simulink model "turtlebot"  (R2023b)
settings: Solver=VariableStepAuto  StartTime=0.0  StopTime=35  RelTol=1e-3
values from neighbouring files (symbols this model uses):
  A = [-2*xcarthography' -2*ycarthography' ones(N,1)]    [circle_linear_regression.m]    (also in turtlebot_sim.m = [r/2 r/2; r/d -r/d])
  Ki = 0.47    [turtlebot_sim.m]
  Kp = 1.2    [turtlebot_sim.m]
  Ts = 0.1    [turtlebot_sim.m]
  x0 = X(1)    [circle_linear_regression.m]    (also in turtlebot_sim.m = [0 0 0])
libraries: slpidlib x2
settings Model: Creator=reda

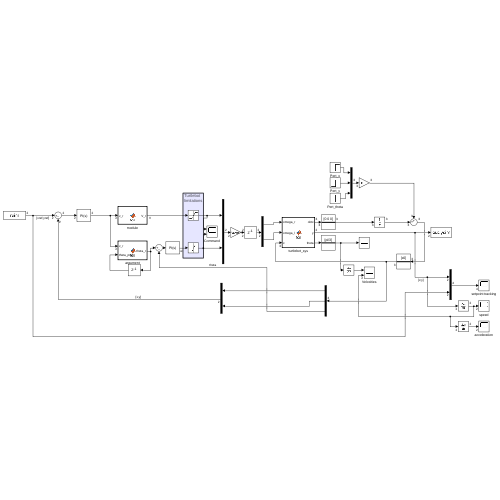
[thumbnail: Simulink's stored preview of the top-level diagram]
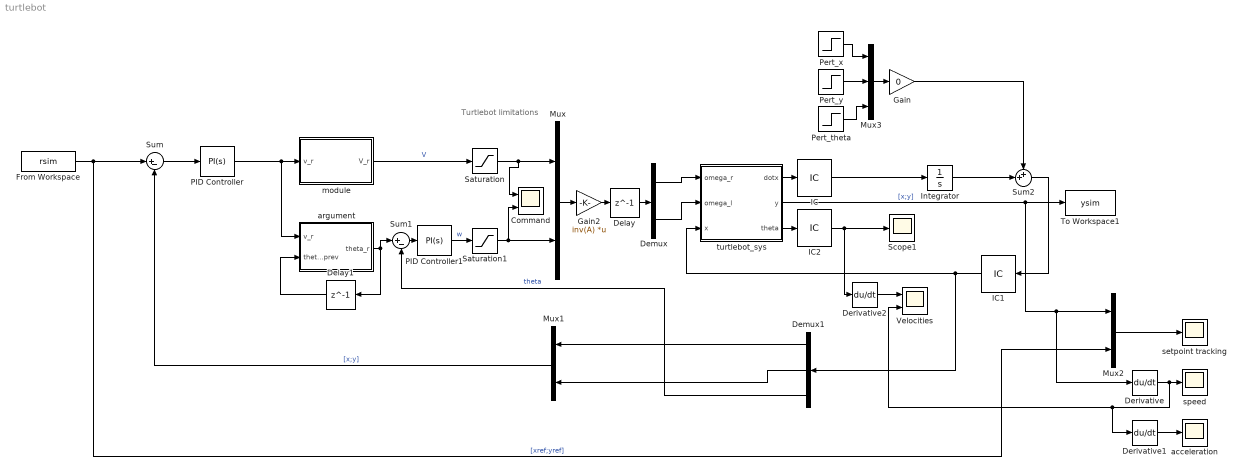
== system turtlebot ==
  note: Turtlebot
      | limitations
  Command : Scope  NumInputPorts=2
  Delay : Delay  DelayLength=1  InitialCondition=0  SampleTime=Ts
  Delay1 : Delay  DelayLength=1  InitialCondition=0  SampleTime=Ts
  Demux : Demux  Outputs=2
  Demux1 : Demux  Outputs=3
  Derivative : Derivative
  Derivative1 : Derivative
  Derivative2 : Derivative
  From Workspace : FromWorkspace  VariableName=rsim
  Gain : Gain  Gain=0
  Gain2 : Gain  Gain=inv(A)  Multiplication=Matrix(K*u) (u vector)
  IC : InitialCondition  Value=[0 0 0]
  IC1 : InitialCondition  Value=x0
  IC2 : InitialCondition  Value=pi/3
  Integrator : Integrator
  Mux : Mux  Inputs=2
  Mux1 : Mux  Inputs=2
  Mux2 : Mux  Inputs=2
  Mux3 : Mux  Inputs=3
  PID Controller : slpidlib/PID Controller  Controller=PI  Form=Parallel  TimeDomain=Continuous-time  UseExternalTs=off  SampleTime=-1  IntegratorMethod=Forward Euler  FilterMethod=Forward Euler  ControllerParametersSource=internal  P=Kp  I=Ki  UseKiTs=off  D=0  N=100  UseFilter=on  TunerSelectOption=Frequency Response Based  InitialConditionSource=internal  InitialConditionForIntegrator=0  InitialConditionForFilter=0  DifferentiatorICPrevScaledInput=0  ExternalReset=none  TrackingMode=off  Kt=1  LimitOutput=off  SatLimitsSource=internal  UpperSaturationLimit=inf  LowerSaturationLimit=-inf  LinearizeAsGain=on  AntiWindupMode=none  Kb=1  LimitIntegrator=off  UpperIntegratorSaturationLimit=inf  LowerIntegratorSaturationLimit=-inf  POutMin=[]  POutMax=[]  IOutMin=[]  IOutMax=[]  DOutMin=[]  DOutMax=[]  NOutMin=[]  NOutMax=[]  SumOutMin=[]  SumOutMax=[]  SaturationOutMin=[]  SaturationOutMax=[]  PParamMin=[]  PParamMax=[]  IParamMin=[]  IParamMax=[]  DParamMin=[]  DParamMax=[]  NParamMin=[]  NParamMax=[]  KbParamMin=[]  KbParamMax=[]  KtParamMin=[]  KtParamMax=[]  KbOutMin=[]  KbOutMax=[]  KtOutMin=[]  KtOutMax=[]  IntegratorOutMin=[]  IntegratorOutMax=[]  FilterOutMin=[]  FilterOutMax=[]  SumI1OutMin=[]  SumI1OutMax=[]  SumI2OutMin=[]  SumI2OutMax=[]  SumI3OutMin=[]  SumI3OutMax=[]  SumI4OutMin=[]  SumI4OutMax=[]  SumDOutMin=[]  SumDOutMax=[]  DifferentiatorOutMin=[]  DifferentiatorOutMax=[]  FilterDiffOutCoefMin=[]  FilterDiffOutCoefMax=[]  ReciprocalOutMin=[]  ReciprocalOutMax=[]  SumDenOutMin=[]  SumDenOutMax=[]  SumNumOutMin=[]  SumNumOutMax=[]  DivideOutMin=[]  DivideOutMax=[]  UdiffTsProdOutMin=[]  UdiffTsProdOutMax=[]  NTsProdOutMin=[]  NTsProdOutMax=[]  UintegralTsProdOutMin=[]  UintegralTsProdOutMax=[]  UngainTsProdOutMin=[]  UngainTsProdOutMax=[]  ClampingZeroOutDataTypeStr=Inherit: Inherit via back propagation  ClampingZeroOutMin=[]  ClampingZeroOutMax=[]  FilterDenConstantOutDataTypeStr=Inherit: Inherit via back propagation  FilterDenConstantOutMin=[]  FilterDenConstantOutMax=[]  PCopyOutDataTypeStr=Inherit: Inherit via back propagation  PCopyOutMin=[]  PCopyOutMax=[]  NCopyOutDataTypeStr=Inherit: Inherit via back propagation  NCopyOutMin=[]  NCopyOutMax=[]  IntegratorContinuousStateAttributes=''  IntegratorStateMustResolveToSignalObject=off  IntegratorRTWStateStorageClass=Auto  FilterContinuousStateAttributes=''  FilterStateMustResolveToSignalObject=off  FilterRTWStateStorageClass=Auto  ParallelPVariant=InternalParameters  IdealPVariant=Disabled  IVariant=InternalParameters  DVariant=Disabled  IntegratorVariant=Continuous  SatVariant=Disabled  AWVariant=Passthrough  PCopyVariant=Disabled  TRVariant=Disabled  FdbkBlocksVariant=Forward  IdealPFdbkVariant=Disabled  SatFdbkVariant=Disabled  DerivativeFilterVariant=Disabled  NVariant=Disabled  NCopyVariant=Disabled_SignalSpec  FilterICVariant=Disabled  IntegratorICVariant=InternalICs  ExternalResetVariant=Disabled  TRSumVariant=Passthrough  SumFdbkVariant=Disabled  SumVariant=Sum_PI  TsampFilterVariant=InternalTs  TsampNgainVariant=Passthrough  TsampIntegralVariant=Disabled_SignalSpec  ExternalSaturationOutDataTypeStr=Inherit: Same as second input
  PID Controller1 : slpidlib/PID Controller  Controller=PI  Form=Parallel  TimeDomain=Continuous-time  UseExternalTs=off  SampleTime=-1  IntegratorMethod=Forward Euler  FilterMethod=Forward Euler  ControllerParametersSource=internal  P=Kp  I=Ki  UseKiTs=off  D=0  N=100  UseFilter=on  TunerSelectOption=Frequency Response Based  InitialConditionSource=internal  InitialConditionForIntegrator=0  InitialConditionForFilter=0  DifferentiatorICPrevScaledInput=0  ExternalReset=none  TrackingMode=off  Kt=1  LimitOutput=off  SatLimitsSource=internal  UpperSaturationLimit=inf  LowerSaturationLimit=-inf  LinearizeAsGain=on  AntiWindupMode=none  Kb=1  LimitIntegrator=off  UpperIntegratorSaturationLimit=inf  LowerIntegratorSaturationLimit=-inf  POutMin=[]  POutMax=[]  IOutMin=[]  IOutMax=[]  DOutMin=[]  DOutMax=[]  NOutMin=[]  NOutMax=[]  SumOutMin=[]  SumOutMax=[]  SaturationOutMin=[]  SaturationOutMax=[]  PParamMin=[]  PParamMax=[]  IParamMin=[]  IParamMax=[]  DParamMin=[]  DParamMax=[]  NParamMin=[]  NParamMax=[]  KbParamMin=[]  KbParamMax=[]  KtParamMin=[]  KtParamMax=[]  KbOutMin=[]  KbOutMax=[]  KtOutMin=[]  KtOutMax=[]  IntegratorOutMin=[]  IntegratorOutMax=[]  FilterOutMin=[]  FilterOutMax=[]  SumI1OutMin=[]  SumI1OutMax=[]  SumI2OutMin=[]  SumI2OutMax=[]  SumI3OutMin=[]  SumI3OutMax=[]  SumI4OutMin=[]  SumI4OutMax=[]  SumDOutMin=[]  SumDOutMax=[]  DifferentiatorOutMin=[]  DifferentiatorOutMax=[]  FilterDiffOutCoefMin=[]  FilterDiffOutCoefMax=[]  ReciprocalOutMin=[]  ReciprocalOutMax=[]  SumDenOutMin=[]  SumDenOutMax=[]  SumNumOutMin=[]  SumNumOutMax=[]  DivideOutMin=[]  DivideOutMax=[]  UdiffTsProdOutMin=[]  UdiffTsProdOutMax=[]  NTsProdOutMin=[]  NTsProdOutMax=[]  UintegralTsProdOutMin=[]  UintegralTsProdOutMax=[]  UngainTsProdOutMin=[]  UngainTsProdOutMax=[]  ClampingZeroOutDataTypeStr=Inherit: Inherit via back propagation  ClampingZeroOutMin=[]  ClampingZeroOutMax=[]  FilterDenConstantOutDataTypeStr=Inherit: Inherit via back propagation  FilterDenConstantOutMin=[]  FilterDenConstantOutMax=[]  PCopyOutDataTypeStr=Inherit: Inherit via back propagation  PCopyOutMin=[]  PCopyOutMax=[]  NCopyOutDataTypeStr=Inherit: Inherit via back propagation  NCopyOutMin=[]  NCopyOutMax=[]  IntegratorContinuousStateAttributes=''  IntegratorStateMustResolveToSignalObject=off  IntegratorRTWStateStorageClass=Auto  FilterContinuousStateAttributes=''  FilterStateMustResolveToSignalObject=off  FilterRTWStateStorageClass=Auto  ParallelPVariant=InternalParameters  IdealPVariant=Disabled  IVariant=InternalParameters  DVariant=Disabled  IntegratorVariant=Continuous  SatVariant=Disabled  AWVariant=Passthrough  PCopyVariant=Disabled  TRVariant=Disabled  FdbkBlocksVariant=Forward  IdealPFdbkVariant=Disabled  SatFdbkVariant=Disabled  DerivativeFilterVariant=Disabled  NVariant=Disabled  NCopyVariant=Disabled_SignalSpec  FilterICVariant=Disabled  IntegratorICVariant=InternalICs  ExternalResetVariant=Disabled  TRSumVariant=Passthrough  SumFdbkVariant=Disabled  SumVariant=Sum_PI  TsampFilterVariant=InternalTs  TsampNgainVariant=Passthrough  TsampIntegralVariant=Disabled_SignalSpec  ExternalSaturationOutDataTypeStr=Inherit: Same as second input
  Pert_theta : Step  Time=180  SampleTime=0
  Pert_x : Step  Time=80  SampleTime=0
  Pert_y : Step  Time=160  SampleTime=0
  Saturation : Saturate  UpperLimit=0.22  LowerLimit=-0.22
  Saturation1 : Saturate  UpperLimit=2.84  LowerLimit=-2.84
  Scope1 : Scope
  Sum : Sum  Inputs=|+-
  Sum1 : Sum  Inputs=|+-
  Sum2 : Sum  Inputs=++|
  To Workspace1 : ToWorkspace  VariableName=ysim  SaveFormat=Structure With Time  SampleTime=-1
  Velocities : Scope  NumInputPorts=2
  acceleration : Scope
  argument : MATLAB Function  TreatAsAtomicUnit=on
  module : MATLAB Function  TreatAsAtomicUnit=on
  setpoint tracking : Scope
  speed : Scope
  turtlebot_sys : MATLAB Function  TreatAsAtomicUnit=on
  wires:
  From Workspace/1 -> Sum/1, Mux2/2  "[xref;yref]"
  module/1(V_r) -> Saturation/1  "V"
  Mux/1 -> Gain2/1
  Demux/1 -> turtlebot_sys/1(omega_r)
  turtlebot_sys/1(dotx) -> IC/1
  argument/1(theta_r) -> Sum1/1, Delay1/1
  Demux1/3 -> Sum1/2  "theta"
  Demux1/1 -> Mux1/1
  Demux1/2 -> Mux1/2
  turtlebot_sys/3(theta) -> IC2/1
  Saturation/1 -> Command/1, Mux/1
  Gain2/1 -> Delay/1
  Delay/1 -> Demux/1
  Mux2/1 -> setpoint tracking/1
  turtlebot_sys/2(y) -> Derivative/1, Mux2/1, To Workspace1/1  "[x;y]"
  Mux1/1 -> Sum/2  "[x;y]"
  PID Controller1/1 -> Saturation1/1  "w"
  Saturation1/1 -> Mux/2, Command/2
  Derivative/1 -> Velocities/2, Derivative1/1, speed/1
  Derivative1/1 -> acceleration/1
  PID Controller/1 -> module/1(v_r), argument/1(v_r)
  Delay1/1 -> argument/2(theta_prev)
  Sum2/1 -> IC1/1
  Pert_x/1 -> Mux3/1
  Pert_y/1 -> Mux3/2
  Pert_theta/1 -> Mux3/3
  Mux3/1 -> Gain/1
  Gain/1 -> Sum2/1
  Integrator/1 -> Sum2/2
  IC/1 -> Integrator/1
  Derivative2/1 -> Velocities/1
  IC2/1 -> Scope1/1, Derivative2/1
  IC1/1 -> turtlebot_sys/3(x), Demux1/1
  Demux/2 -> turtlebot_sys/2(omega_l)
  Sum/1 -> PID Controller/1
  Sum1/1 -> PID Controller1/1

== matlab function turtlebot/module ==
  data: v_r input; V_r output
function V_r  = fcn(v_r)
V_r = sqrt(v_r(1)^2+v_r(2)^2);

== matlab function turtlebot/argument ==
  data: v_r input; theta_r output; theta_prev input
function theta_r  = fcn(v_r, theta_prev)

%We use atan2() and not atan() because atan(x) -> [-pi/2; pi/2] and atan2 -> [0;2pi]
%We work at 360° so we must use atan2
theta=wrapTo2Pi(atan2(v_r(2),v_r(1)));

%Sometimes, there may be a jump between (2pi - delta) rad  and 0rad so the
%robots thinks he has to turn back (2pi-delta) rad instead of just rotate
%by delta rad. (delta being a tiny angle)
%That's why we have to unwrap the angle with the previous angle so that the
%difference between the previous angle and the current angle is not greater
%than pi
unwrapped_theta = unwrap([theta_prev theta]);

theta_r=unwrapped_theta(2);

== matlab function turtlebot/turtlebot_sys ==
  data: omega_r input; dotx output; omega_l input; x input; y output; theta output
function [dotx, y, theta]  = fcn(omega_r,omega_l, x)
dotx=[(33e-3*(omega_r+omega_l)/2)*cos(x(3)); (33e-3*(omega_r+omega_l)/2)*sin(x(3)); 33e-3/160e-3*(omega_r-omega_l)];
y= [x(1); x(2)];
theta = x(3);
